simulink model "practica1validacion"  (R2019b)
settings: Solver=VariableStepAuto  StartTime=0.0  StopTime=10.0  RelTol=1e-3
settings Model: Creator=Usuario  LastModifiedBy=Usuario

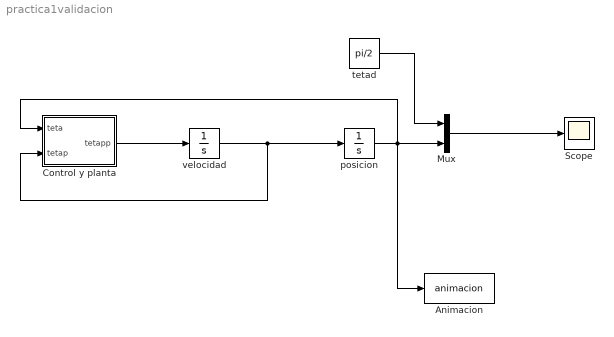
== system practica1validacion ==
  "Animacion " : MATLABFcn  MATLABFcn=animacion  OutputDimensions=0
  Control y planta : MATLAB Function  TreatAsAtomicUnit=on
  Mux : Mux  Inputs=2
  Scope : Scope
  posicion : Integrator
  tetad : Constant  Value=pi/2
  velocidad : Integrator
  wires:
  Control y planta/1(tetapp) -> velocidad/1
  velocidad/1 -> Control y planta/2(tetap), posicion/1
  posicion/1 -> "Animacion "/1, Control y planta/1(teta), Mux/2
  tetad/1 -> Mux/1
  Mux/1 -> Scope/1

== matlab function practica1validacion/Control y planta ==
  data: teta input; tetapp output; tetap input
function tetapp = fcn(teta,tetap)
%%parametros
m = 1;
lc = 0.5;
I = 1;
g = 9.81;
B=0.003;
kp = 450;
kd = 10;
tetad=pi/2;
%control
e=tetad-teta;
tau = kp*e-kd*tetap;
%planta
tetapp = 1/(m*lc^2+I)*(tau-m*g*lc*sin(teta)-B*tetap);
